simulink model "ITMBS_square_M2_Test_harness"  (R2023a)
settings: Solver=FixedStepDiscrete  StartTime=0.0  StopTime=18  FixedStep=0.05  RelTol=1e-3  EnableMultiTasking=on
values from neighbouring files (symbols this model uses):
  dist = 100    [M2_square.m]
undefined symbols (not defined in the file or in its folder): sigbuilder_block
libraries: legoev3lib x2
settings Model: ExtModeTrigDuration=2  Creator=3w09  LastModifiedBy=Sachin K S
settings SolverCC: PositivePriorityOrder=on  AutoInsertRateTranBlk=on
settings OptimizationCC: EnhancedBackFolding=on  PassReuseOutputArgsAs=Individual arguments  ZeroExternalMemoryAtStartup=off  ZeroInternalMemoryAtStartup=off  MaxStackSize=64  OptimizeBlockOrder=speed  DifferentSizesBufferReuse=on  OptimizationCustomize=off  EfficientTunableParamExpr=on
settings DebuggingCC: ParameterTunabilityLossMsg=error
settings HardwareCC: ProdBitPerPointer=32  ProdBitPerSizeT=32  ProdBitPerPtrDiffT=32  ProdLargestAtomicInteger=Long  ProdWordSize=32  ProdHWDeviceType=ARM Compatible->ARM 9  UseEmbeddedCoderFeatures=off  UseSimulinkCoderFeatures=off
settings SFSimCC: MATLABDynamicMemAlloc=off
settings RTWCC: Description=Embedded Coder  SystemTargetFile=ert.tlc  HardwareBoard=LEGO MINDSTORMS EV3  TLCOptions="-aInlineSetEventsForThisBaseRateFcn=TLC_FALSE -aSuppressMultiTaskScheduler=TLC_FALSE  -aRateBasedStepFcn=0"  TemplateMakefile=ert_default_tmf  Toolchain=Sourcery G++ Lite v2009q3
settings CodeAppCC: ForceParamTrailComments=on  IgnoreCustomStorageClasses=off  OperatorAnnotations=on  SimulinkDataObjDesc=on  SFDataObjDesc=on  InsertBlockDesc=on
settings ERTTargetCC: SupportContinuousTime=on  SupportNonInlinedSFcns=on  SupportVariableSizeSignals=on  ExtModeTransport=2  ExtModeStaticAlloc=on  ExtModeMexFile=ext_xcp  ExtModeIntrfLevel=Level2 - Open

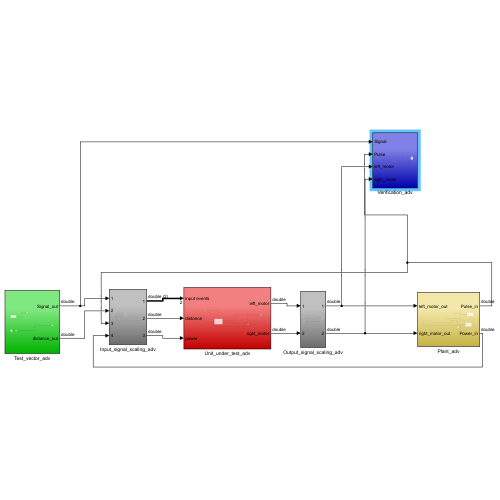
[thumbnail: Simulink's stored preview of the top-level diagram]
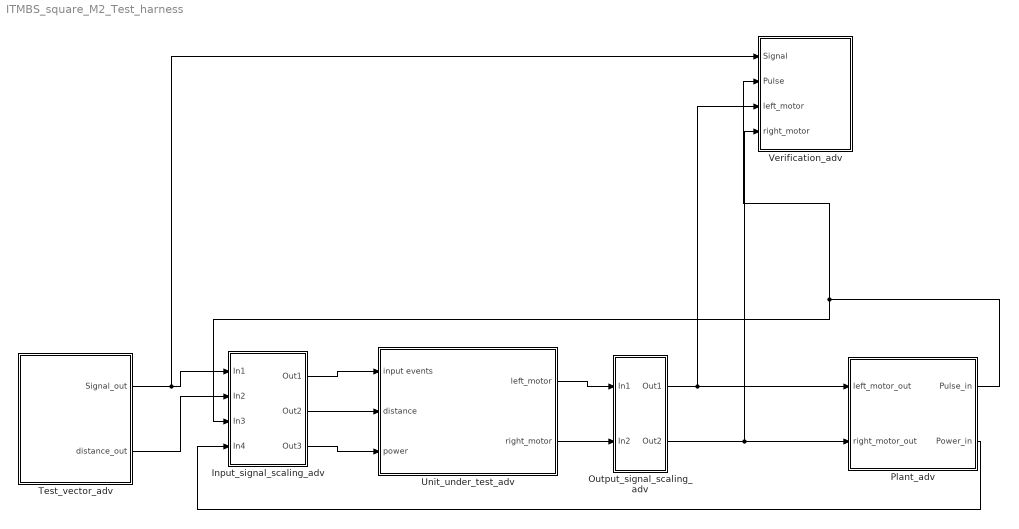
== system ITMBS_square_M2_Test_harness ==
  Input_signal_scaling_adv : Subsystem
  Output_signal_scaling_adv : Subsystem
  Plant_adv : Subsystem
  Test_vector_adv : Subsystem
  Unit_under_test_adv : Subsystem
  Verification_adv : Subsystem
  wires:
  Unit_under_test_adv/1(left_motor) -> Output_signal_scaling_adv/1(In1)
  Unit_under_test_adv/2(right_motor) -> Output_signal_scaling_adv/2(In2)
  Input_signal_scaling_adv/1(Out1) -> Unit_under_test_adv/1(input events)
  Test_vector_adv/1(Signal_out) -> Verification_adv/1(Signal), Input_signal_scaling_adv/1(In1)
  Input_signal_scaling_adv/3(Out3) -> Unit_under_test_adv/3(power)
  Input_signal_scaling_adv/2(Out2) -> Unit_under_test_adv/2(distance)
  Test_vector_adv/2(distance_out) -> Input_signal_scaling_adv/2(In2)
  Output_signal_scaling_adv/1(Out1) -> Plant_adv/1(left_motor_out), Verification_adv/3(left_motor)
  Output_signal_scaling_adv/2(Out2) -> Verification_adv/4(right_motor), Plant_adv/2(right_motor_out)
  Plant_adv/1(Pulse_in) -> Verification_adv/2(Pulse), Input_signal_scaling_adv/3(In3)
  Plant_adv/2(Power_in) -> Input_signal_scaling_adv/4(In4)

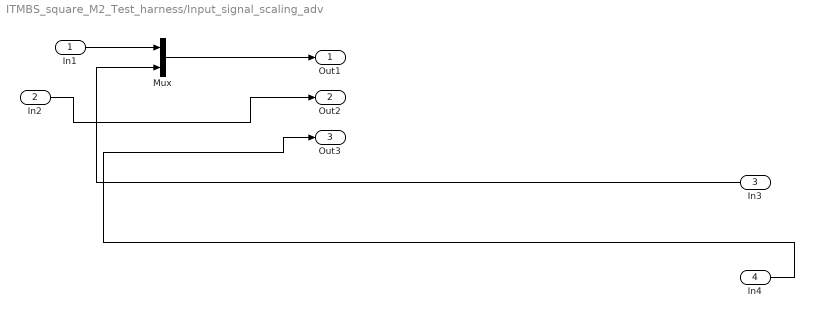
== system ITMBS_square_M2_Test_harness/Input_signal_scaling_adv ==
  In1 : Inport
  In2 : Inport  Port=2
  In3 : Inport  Port=3
  In4 : Inport  Port=4
  Mux : Mux  Inputs=2
  Out1 : Outport
  Out2 : Outport  Port=2
  Out3 : Outport  Port=3
  wires:
  In3/1 -> Mux/2
  In4/1 -> Out3/1
  In2/1 -> Out2/1
  Mux/1 -> Out1/1
  In1/1 -> Mux/1

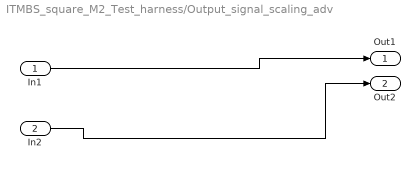
== system ITMBS_square_M2_Test_harness/Output_signal_scaling_adv ==
  In1 : Inport
  In2 : Inport  Port=2
  Out1 : Outport
  Out2 : Outport  Port=2
  wires:
  In2/1 -> Out2/1
  In1/1 -> Out1/1

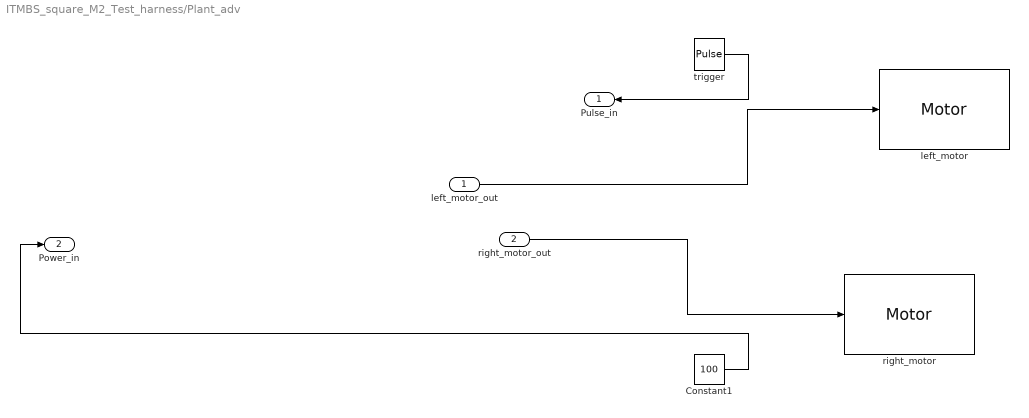
== system ITMBS_square_M2_Test_harness/Plant_adv ==
  left_motor_out : Inport
  right_motor_out : Inport  Port=2
  Constant1 : Constant  Value=100
  left_motor : legoev3lib/Motor  sportNumber=B  sstopAction=Brake
  right_motor : legoev3lib/Motor  sportNumber=A  sstopAction=Brake
  trigger : DiscretePulseGenerator  Period=3  PulseWidth=2  SampleTime=0.05
  Pulse_in : Outport
  Power_in : Outport  Port=2
  wires:
  right_motor_out/1 -> right_motor/1
  trigger/1 -> Pulse_in/1
  Constant1/1 -> Power_in/1
  left_motor_out/1 -> left_motor/1

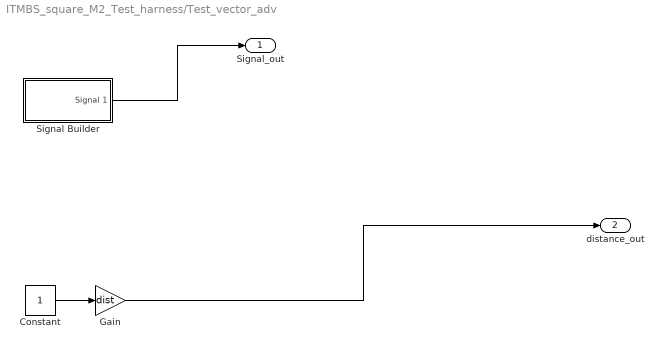
== system ITMBS_square_M2_Test_harness/Test_vector_adv ==
  Constant : Constant
  Gain : Gain  Gain=dist
  Signal Builder : Subsystem  Tag=STV Subsys  LoadFcn=sigbuilder_block('load');  StartFcn=sigbuilder_block('start');  StopFcn=sigbuilder_block('stop');  ClipboardFcn=sigbuilder_block('clipboard');  mask(Sigbuilder block){tuvar=[0:10]}
      mask help: Simulink:masks:SigbuilderBlock_MD
      mask init:
      | if ~strcmp(get_param(bdroot(gcbh),'SimulationStatus'),'stopped') tuvar = sigbuilder_block('maskInit'); end
      settings: CopyFcn=sigbuilder_block('copy');  DeleteFcn=sigbuilder_block('delete');  ModelCloseFcn=sigbuilder_block('modelClose');  PreSaveFcn=sigbuilder_block('preSave');  PauseFcn=sigbuilder_block('pause');  ContinueFcn=sigbuilder_block('continue');  NameChangeFcn=sigbuilder_block('namechange');  OpenFcn=sigbuilder_block('open',[6 30 1012.5 447.75 ]);  CloseFcn=sigbuilder_block('close');
      mask Display: plot(0, 0, 100, 100,[2, 2, 32, 32, 2], [68, 8, 8, 68, 68],[32, 2], [38, 38], [32, 19, 2],[53, 60, 44], [32, 17, 17, 2],[16, 16, 31, 31]);txt = getActiveGroup(gcbh);text(2, 100, txt,'verticalAlignment', 'top');
  Signal_out : Outport
  distance_out : Outport  Port=2
  wires:
  Constant/1 -> Gain/1
  Gain/1 -> distance_out/1
  Signal Builder/1(Signal 1) -> Signal_out/1

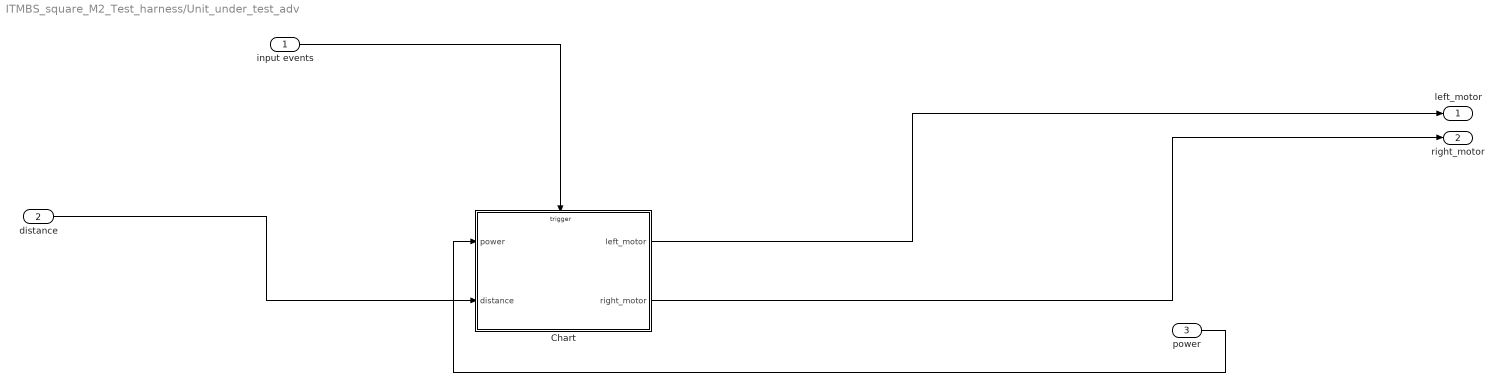
== system ITMBS_square_M2_Test_harness/Unit_under_test_adv ==
  input events : Inport
  distance : Inport  Port=2
  power : Inport  Port=3
  Chart : Stateflow chart  TreatAsAtomicUnit=on
  left_motor : Outport
  right_motor : Outport  Port=2
  wires:
  Chart/2(right_motor) -> right_motor/1
  Chart/1(left_motor) -> left_motor/1
  distance/1 -> Chart/2(distance)
  input events/1 -> Chart/Trigger
  power/1 -> Chart/1(power)

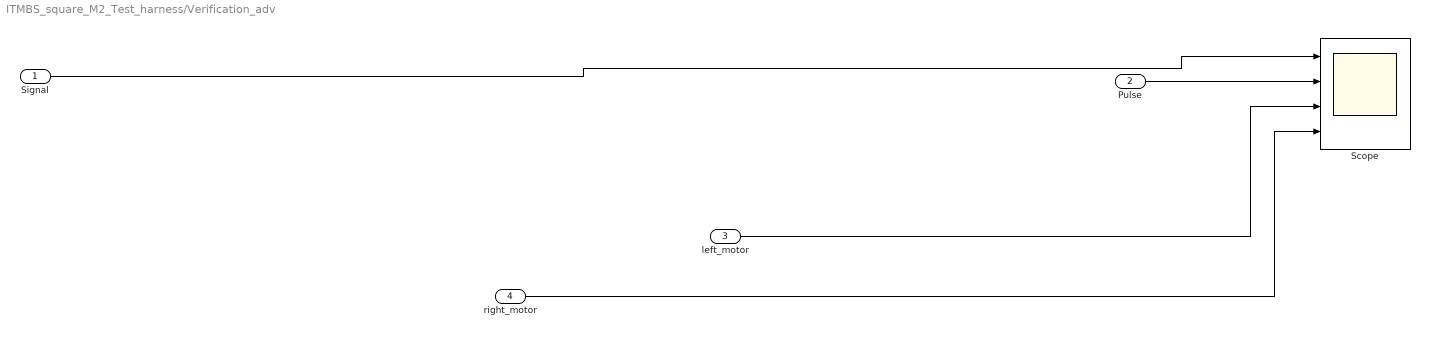
== system ITMBS_square_M2_Test_harness/Verification_adv ==
  Signal : Inport
  Pulse : Inport  Port=2
  left_motor : Inport  Port=3
  right_motor : Inport  Port=4
  Scope : Scope  NumInputPorts=4
  wires:
  Signal/1 -> Scope/1
  left_motor/1 -> Scope/3
  right_motor/1 -> Scope/4
  Pulse/1 -> Scope/2

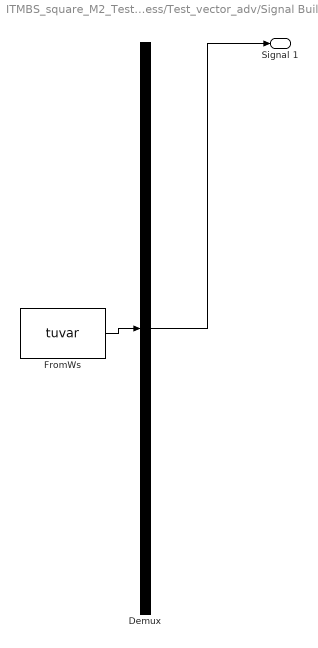
== system ITMBS_square_M2_Test_harness/Test_vector_adv/Signal Builder ==
  Demux : Demux  Tag=STV Demux  Outputs=1
      settings: DisplayOption=none
  FromWs : FromWorkspace  Tag=STV FromWs  VariableName=tuvar
      SigBuilderData=|
      | common.afterFinalStr = 'Extrapolate'
      | common.sampleTime = 0
      | dataSet.timeRange = [0 10]
      | dataSet.name = 'Group 1'
      | sbobj.Groups.Name = 'Group 1'
      | sbobj.Groups.Signals.Name = 'Signal 1'
      | sbobj.Groups.Signals.XData = [0 2.02 2.02 3.02 3.02 7 7 7.8 7.8 8.18 8.18 9 9 10]
      | sbobj.Groups.Signals.YData = [0 0 1 1 0 -0.005 0.995 1 0 0 0.995 0.995 0 0]
  Signal 1 : Outport  Tag=STV Outport
  wires:
  Demux/1 -> Signal 1/1
  FromWs/1 -> Demux/1

== stateflow chart ITMBS_square_M2_Test_harness/Unit_under_test_adv/Chart ==
  settings: executeAtInitialization=1
  state OFF_sq
    entry:
    right_motor=0;
    left_motor=0;
    c=0;
  state ON_sq
    right_motor =power;
    left_motor =power;
  state sq
    entry:
    right_motor= 0;
    left_motor=power;
  (default) -> ON_sq
  ON_sq -> OFF_sq [order 1] : [pushbutton_event_input]
  sq -> ON_sq [order 2] : [after(0.32,sec)]
  OFF_sq -> (junction 36)
  sq -> OFF_sq [order 1] : [pushbutton_event_input]
  ON_sq -> sq [order 2] : [after(0.0192* distance ,sec)]
  (junction 38) -> ON_sq [order 1] : [c==2]
  (junction 36) -> (junction 37) [order 1] : [pushbutton_event_input]
  (junction 36) -> (junction 38) [order 2]
  (junction 37) -> (junction 39) : {c= c+1;}
  (junction 39) -> (junction 38)
  (junction 38) -> (junction 53) [order 2]
  data: power input; c local; left_motor output; right_motor output; distance input
  events: pushbutton_event_input input RISING_EDGE_EVENT; trigger input RISING_EDGE_EVENT
